simulink model "ukl_reg_I"  (R2023a)
settings: Solver=VariableStepAuto  StartTime=0.0  StopTime=300.0  RelTol=1e-3
undefined symbols (not defined in the file): h, SP, T, tau
settings Model: Creator=jpawl  LastModifiedBy=jpawl

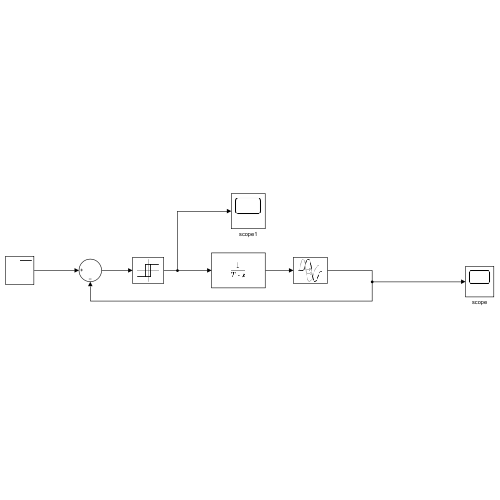
[thumbnail: Simulink's stored preview of the top-level diagram]
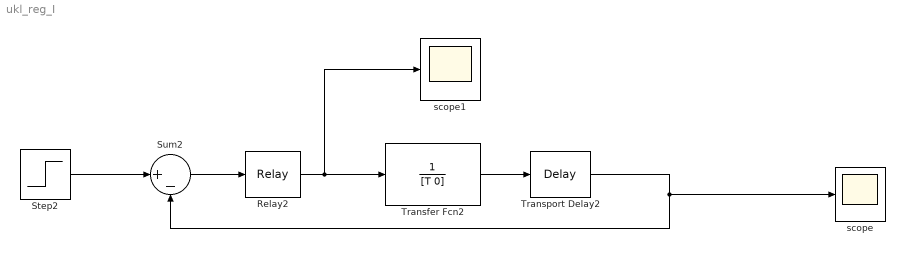
== system ukl_reg_I ==
  Relay2 : Relay  OnSwitchValue=h  OffSwitchValue=-h  OffOutputValue=-1
  Step2 : Step  After=SP  SampleTime=0
  Sum2 : Sum  Inputs=|+-
  Transfer Fcn2 : TransferFcn  Denominator=[T 0]
  Transport Delay2 : TransportDelay  DelayTime=tau  PadeOrder=10
  scope : Scope
  scope1 : Scope
  wires:
  Relay2/1 -> Transfer Fcn2/1, scope1/1
  Transfer Fcn2/1 -> Transport Delay2/1
  Step2/1 -> Sum2/1
  Sum2/1 -> Relay2/1
  Transport Delay2/1 -> scope/1, Sum2/2
